simulink model "SignalModelL6_shim_a"  (R2017a)
settings: Solver=FixedStepAuto  StartTime=0.0  StopTime=20  FixedStep=0.01  RelTol=1e-3
undefined symbols (not defined in the file): p2
settings Model: Creator=roman  LastModifiedBy=roman

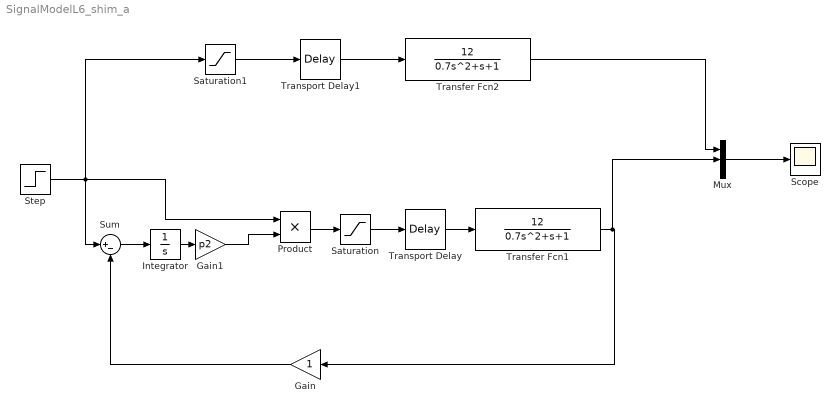
== system SignalModelL6_shim_a ==
  Gain : Gain
  Gain1 : Gain  Gain=p2
  Integrator : Integrator
  Mux : Mux  Inputs=3
  Product : Product
  Saturation : Saturate  UpperLimit=2000  LowerLimit=-2000
  Saturation1 : Saturate  UpperLimit=2000  LowerLimit=-2000
  Scope : Scope
  Step : Step  Time=0  SampleTime=0
  Sum : Sum  Inputs=|+-
  Transfer Fcn1 : TransferFcn  Numerator=[12]  Denominator=[0.7 1 1]
  Transfer Fcn2 : TransferFcn  Numerator=[12]  Denominator=[0.7 1 1]
  Transport Delay : TransportDelay  DelayTime=0.1
  Transport Delay1 : TransportDelay  DelayTime=0.1
  wires:
  Saturation1/1 -> Transport Delay1/1
  Mux/1 -> Scope/1
  Step/1 -> Product/1, Sum/1, Saturation1/1
  Transfer Fcn2/1 -> Mux/1
  Gain/1 -> Sum/2
  Transfer Fcn1/1 -> Mux/2, Gain/1
  Saturation/1 -> Transport Delay/1
  Transport Delay/1 -> Transfer Fcn1/1
  Transport Delay1/1 -> Transfer Fcn2/1
  Product/1 -> Saturation/1
  Gain1/1 -> Product/2
  Integrator/1 -> Gain1/1
  Sum/1 -> Integrator/1
